simulink library "Hqaud_model_LIB_SI"  (Simulink 7.8)
settings: Solver=ode45  StartTime=0.0  StopTime=10.0  RelTol=1e-3
values from neighbouring files (symbols this model uses):
  g = 9.8065    [kostas_malakies.mat]    (also in kostas_malakies2.mat; load_PMModel.m = 9.81; main_last.m; matlab.mat)
  mass = 0.66    [kostas_malakies.mat]    (also in kostas_malakies2.mat; load_PMModel.m = 0.687; main_last.m)
  pitch_cmd2pitch_1stOrd = 1.42468924998    [kostas_malakies.mat]    (also in kostas_malakies2.mat)
  roll_cmd2roll_1stOrd = 1.38101661575    [kostas_malakies.mat]    (also in kostas_malakies2.mat)
  Td_pitch_1stOrd = 0.0601685534007    [kostas_malakies.mat]    (also in kostas_malakies2.mat)
  Td_pitch_2ndOrd = 0.0464096828042    [kostas_malakies.mat]    (also in kostas_malakies2.mat)
  Td_roll_1stOrd = 0.0529497254218    [kostas_malakies.mat]    (also in kostas_malakies2.mat)
  Td_roll_2ndOrd = 0.0402297098443    [kostas_malakies.mat]    (also in kostas_malakies2.mat)
  Td_thrust_0thOrd = 0.041    [kostas_malakies.mat]    (also in kostas_malakies2.mat)
  Td_yaw_1stOrd = 0.110660814834    [kostas_malakies.mat]    (also in kostas_malakies2.mat)
  thrust_cmd2thrust_0thOrd = 0.876575459522    [kostas_malakies.mat]    (also in kostas_malakies2.mat)
  THRUST_CMD_GAIN = -0.0835    [kostas_malakies.mat]    (also in kostas_malakies2.mat; load_PMModel.m)
  yaw_cmd2yaw_1stOrd = 2.01792090263    [kostas_malakies.mat]    (also in kostas_malakies2.mat)
libraries: cstblocks x6, Hqaud_model_LIB_SI x5, dspnetwork x2, simulink x1
settings Model: Creator=andi  LastModifiedBy=burrimi

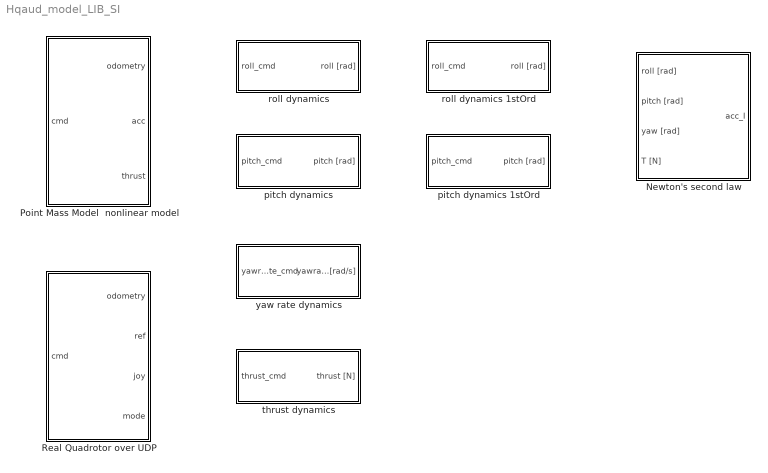
== system Hqaud_model_LIB_SI ==
  "Newton's second law  " : Subsystem
  Point Mass Model  nonlinear model : Subsystem
  Real Quadrotor over UDP : Subsystem
  "pitch dynamics  " : Subsystem
  pitch dynamics 1stOrd : Subsystem
  roll dynamics : Subsystem
  roll dynamics 1stOrd : Subsystem
  "thrust dynamics  " : Subsystem
  "yaw rate dynamics  " : Subsystem

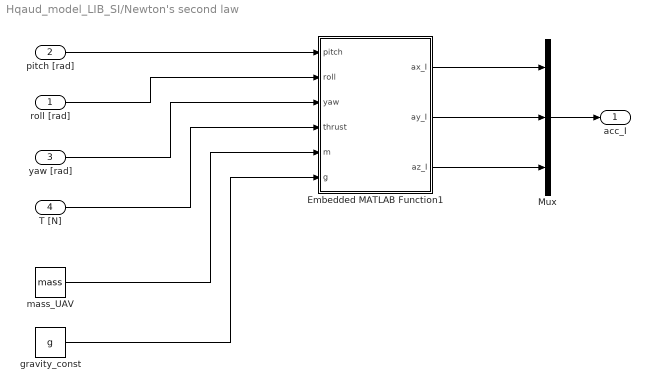
== system Hqaud_model_LIB_SI/Newton's second law   ==
  "roll [rad]  " : Inport  PortDimensions=1
  "pitch [rad]  " : Inport  Port=2  PortDimensions=1
  "yaw [rad]  " : Inport  Port=3  PortDimensions=1
  T [N] : Inport  Port=4  PortDimensions=1
  Embedded MATLAB Function1 : MATLAB Function  TreatAsAtomicUnit=on
  Mux : Mux  Inputs=3
  gravity_const : Constant  Value=g
  mass_UAV : Constant  Value=mass
  "acc_I  " : Outport  PortDimensions=3
  wires:
  Embedded MATLAB Function1/1(ax_I) -> Mux/1
  Embedded MATLAB Function1/2(ay_I) -> Mux/2
  Embedded MATLAB Function1/3(az_I) -> Mux/3
  Mux/1 -> "acc_I  "/1
  "pitch [rad]  "/1 -> Embedded MATLAB Function1/1(pitch)
  "roll [rad]  "/1 -> Embedded MATLAB Function1/2(roll)
  "yaw [rad]  "/1 -> Embedded MATLAB Function1/3(yaw)
  T [N]/1 -> Embedded MATLAB Function1/4(thrust)
  mass_UAV/1 -> Embedded MATLAB Function1/5(m)
  gravity_const/1 -> Embedded MATLAB Function1/6(g)

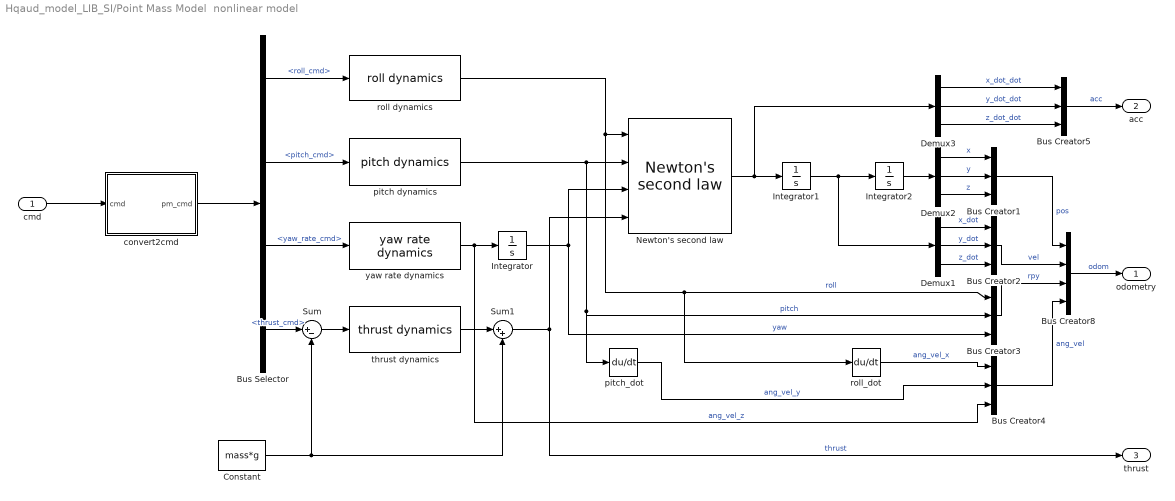
== system Hqaud_model_LIB_SI/Point Mass Model  nonlinear model ==
  cmd : Inport
  Bus Creator{1..5} (5 alike) : BusCreator  Inputs=3
  Bus Creator8 : BusCreator
  Bus Selector : BusSelector  OutputSignals=roll_cmd,pitch_cmd,yaw_rate_cmd,thrust_cmd
  Constant : Constant  Value=mass*g
  Demux1 : Demux  Outputs=3
  Demux2 : Demux  Outputs=3
  Demux3 : Demux  Outputs=3
  Integrator : Integrator
  Integrator1 : Integrator
  Integrator2 : Integrator
  "Newton's second law  " : Hqaud_model_LIB_SI/Newton's second law    SystemSampleTime=-1
  Sum : Sum  Inputs=|+-
  Sum1 : Sum  Inputs=|++
  convert2cmd : Subsystem
  "pitch dynamics  " : Hqaud_model_LIB_SI/pitch dynamics    SystemSampleTime=-1
  pitch_dot : Derivative
  roll dynamics : Hqaud_model_LIB_SI/roll dynamics  SystemSampleTime=-1
  roll_dot : Derivative
  "thrust dynamics  " : Hqaud_model_LIB_SI/thrust dynamics    SystemSampleTime=-1
  "yaw rate dynamics  " : Hqaud_model_LIB_SI/yaw rate dynamics    SystemSampleTime=-1
  odometry : Outport
  acc : Outport  Port=2
  "thrust   " : Outport  Port=3  PortDimensions=1
  wires:
  pitch_dot/1 -> Bus Creator4/2  "ang_vel_y"
  roll_dot/1 -> Bus Creator4/1  "ang_vel_x"
  Sum1/1 -> "thrust   "/1, "Newton's second law  "/4  "thrust"
  Demux3/3 -> Bus Creator5/3  "z_dot_dot"
  Demux3/2 -> Bus Creator5/2  "y_dot_dot"
  Demux3/1 -> Bus Creator5/1  "x_dot_dot"
  Bus Creator5/1 -> acc/1  "acc"
  Demux1/3 -> Bus Creator2/3  "z_dot"
  Demux1/2 -> Bus Creator2/2  "y_dot"
  Demux1/1 -> Bus Creator2/1  "x_dot"
  Demux2/1 -> Bus Creator1/1  "x"
  Demux2/3 -> Bus Creator1/3  "z"
  Bus Creator8/1 -> odometry/1  "odom"
  Bus Creator1/1 -> Bus Creator8/1  "pos"
  Bus Creator2/1 -> Bus Creator8/2  "vel"
  Bus Creator3/1 -> Bus Creator8/3  "rpy"
  Bus Creator4/1 -> Bus Creator8/4  "ang_vel"
  Bus Selector/3 -> "yaw rate dynamics  "/1  "<yaw_rate_cmd>"
  Bus Selector/2 -> "pitch dynamics  "/1  "<pitch_cmd>"
  cmd/1 -> convert2cmd/1(cmd)
  Bus Selector/4 -> Sum/1  "<thrust_cmd>"
  Sum/1 -> "thrust dynamics  "/1
  Constant/1 -> Sum1/2, Sum/2
  Demux2/2 -> Bus Creator1/2  "y"
  Integrator2/1 -> Demux2/1
  Integrator1/1 -> Demux1/1, Integrator2/1
  "Newton's second law  "/1 -> Demux3/1, Integrator1/1
  roll dynamics/1 -> roll_dot/1, Bus Creator3/1, "Newton's second law  "/1  "roll"
  "pitch dynamics  "/1 -> pitch_dot/1, Bus Creator3/2, "Newton's second law  "/2  "pitch"
  "thrust dynamics  "/1 -> Sum1/1
  Integrator/1 -> Bus Creator3/3, "Newton's second law  "/3  "yaw"
  "yaw rate dynamics  "/1 -> Bus Creator4/3, Integrator/1  "ang_vel_z"
  Bus Selector/1 -> roll dynamics/1  "<roll_cmd>"
  convert2cmd/1(pm_cmd) -> Bus Selector/1

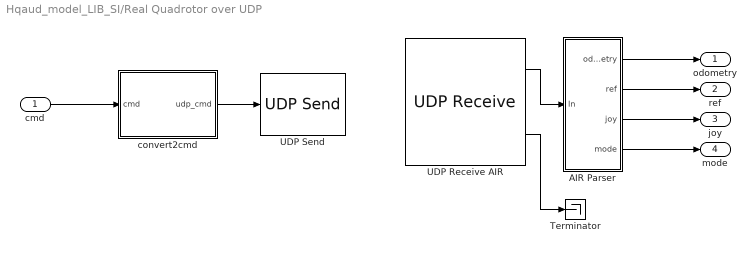
== system Hqaud_model_LIB_SI/Real Quadrotor over UDP ==
  cmd : Inport
  AIR Parser : Subsystem
  Terminator : Terminator
  UDP Receive AIR : dspnetwork/UDP Receive  localURL='0.0.0.0'  localPort=9590  remoteURL='127.0.0.1'  remotePort=-1  recvBufferSize=8192  dims=30  signalDatatype=single  isVarSize=off  showBlockingTime=on  blockingTime=0.5  sampletime=Ts  blockPlatform=LINUX
  UDP Send : dspnetwork/UDP Send  remoteURL='127.0.0.1'  remotePort=9091  localURL='255.255.255.255'  localPortSource=Automatically determine  localPort=-1  sampletime=-1  blockPlatform=LINUX  separateLengthPort=0
  convert2cmd : Subsystem
  odometry : Outport
  ref : Outport  Port=2
  joy : Outport  Port=3
  "mode   " : Outport  Port=4  PortDimensions=1
  wires:
  cmd/1 -> convert2cmd/1(cmd)
  convert2cmd/1(udp_cmd) -> UDP Send/1
  UDP Receive AIR/1 -> AIR Parser/1(In)
  AIR Parser/1(odometry) -> odometry/1
  AIR Parser/2(ref) -> ref/1
  AIR Parser/3(joy) -> joy/1
  AIR Parser/4(mode) -> "mode   "/1
  UDP Receive AIR/2 -> Terminator/1

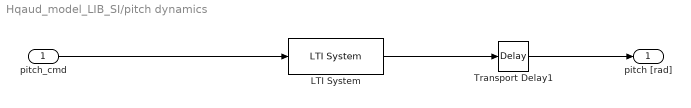
== system Hqaud_model_LIB_SI/pitch dynamics   ==
  "pitch_cmd  " : Inport  PortDimensions=1
  LTI System : cstblocks/LTI System  SystemSampleTime=-1  sys=dynamics_pitch_2ndOrd  IC=[]
  Transport Delay1 : TransportDelay  DelayTime=Td_pitch_2ndOrd  PadeOrder=delay_pade_order
  "pitch [rad] " : Outport  PortDimensions=1
  wires:
  LTI System/1 -> Transport Delay1/1
  "pitch_cmd  "/1 -> LTI System/1
  Transport Delay1/1 -> "pitch [rad] "/1

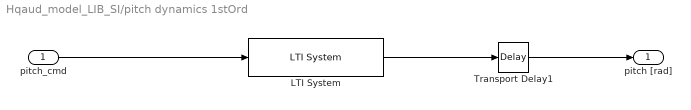
== system Hqaud_model_LIB_SI/pitch dynamics 1stOrd ==
  "pitch_cmd  " : Inport  PortDimensions=1
  LTI System : cstblocks/LTI System  SystemSampleTime=-1  sys=dynamics_pitch_1stOrd  IC=[]
  Transport Delay1 : TransportDelay  DelayTime=Td_pitch_1stOrd  PadeOrder=delay_pade_order
  "pitch [rad] " : Outport  PortDimensions=1
  wires:
  Transport Delay1/1 -> "pitch [rad] "/1
  "pitch_cmd  "/1 -> LTI System/1
  LTI System/1 -> Transport Delay1/1

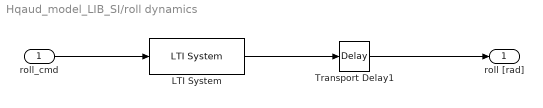
== system Hqaud_model_LIB_SI/roll dynamics ==
  "roll_cmd  " : Inport  PortDimensions=1
  LTI System : cstblocks/LTI System  SystemSampleTime=-1  sys=dynamics_roll_2ndOrd  IC=[]
  Transport Delay1 : TransportDelay  DelayTime=Td_roll_2ndOrd  PadeOrder=delay_pade_order
  "roll [rad]  " : Outport  PortDimensions=1
  wires:
  LTI System/1 -> Transport Delay1/1
  Transport Delay1/1 -> "roll [rad]  "/1
  "roll_cmd  "/1 -> LTI System/1

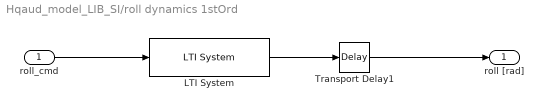
== system Hqaud_model_LIB_SI/roll dynamics 1stOrd ==
  "roll_cmd  " : Inport  PortDimensions=1
  LTI System : cstblocks/LTI System  SystemSampleTime=-1  sys=dynamics_roll_1stOrd  IC=[]
  Transport Delay1 : TransportDelay  DelayTime=Td_roll_1stOrd  PadeOrder=delay_pade_order
  "roll [rad]  " : Outport  PortDimensions=1
  wires:
  "roll_cmd  "/1 -> LTI System/1
  Transport Delay1/1 -> "roll [rad]  "/1
  LTI System/1 -> Transport Delay1/1

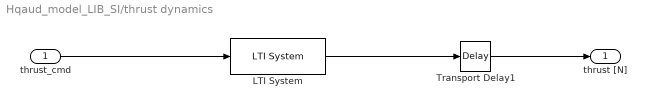
== system Hqaud_model_LIB_SI/thrust dynamics   ==
  "thrust_cmd  " : Inport  PortDimensions=1
  LTI System : cstblocks/LTI System  SystemSampleTime=-1  sys=dynamics_thrust_0thOrd  IC=[]
  Transport Delay1 : TransportDelay  DelayTime=Td_thrust_0thOrd  PadeOrder=delay_pade_order
  "thrust [N] " : Outport  PortDimensions=1
  wires:
  LTI System/1 -> Transport Delay1/1
  Transport Delay1/1 -> "thrust [N] "/1
  "thrust_cmd  "/1 -> LTI System/1

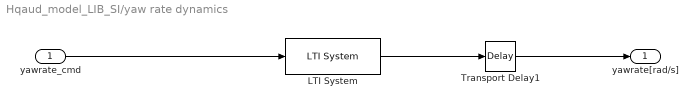
== system Hqaud_model_LIB_SI/yaw rate dynamics   ==
  "yawrate_cmd  " : Inport  PortDimensions=1
  LTI System : cstblocks/LTI System  SystemSampleTime=-1  sys=dynamics_yaw_1stOrd  IC=[]
  Transport Delay1 : TransportDelay  DelayTime=Td_yaw_1stOrd
  "yawrate[rad/s] " : Outport  PortDimensions=1
  wires:
  LTI System/1 -> Transport Delay1/1
  Transport Delay1/1 -> "yawrate[rad/s] "/1
  "yawrate_cmd  "/1 -> LTI System/1

== system Hqaud_model_LIB_SI/Point Mass Model  nonlinear model/convert2cmd ==
  cmd : Inport
  Bus Creator8 : BusCreator
  Bus Selector : BusSelector  OutputSignals=pitch_cmd,roll_cmd,thrust_cmd,yaw_rate_cmd
  pm_cmd : Outport
  wires:
  Bus Creator8/1 -> pm_cmd/1
  cmd/1 -> Bus Selector/1
  Bus Selector/1 -> Bus Creator8/1  "<pitch_cmd>"
  Bus Selector/2 -> Bus Creator8/2  "<roll_cmd>"
  Bus Selector/4 -> Bus Creator8/4  "<yaw_rate_cmd>"
  Bus Selector/3 -> Bus Creator8/3  "<thrust_cmd>"

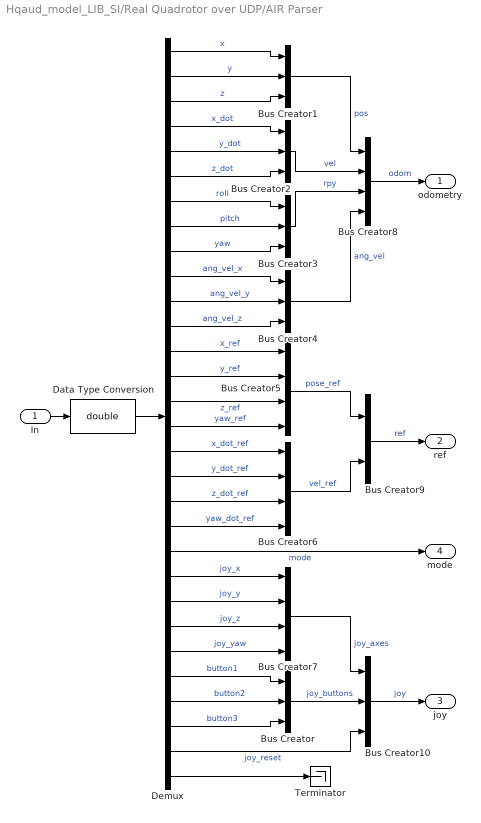
== system Hqaud_model_LIB_SI/Real Quadrotor over UDP/AIR Parser ==
  In : Inport
  Bus Creator{,1..4,10} (6 alike) : BusCreator  Inputs=3
  Bus Creator{5..8} (4 alike) : BusCreator
  Bus Creator9 : BusCreator  Inputs=2
  Data Type Conversion : DataTypeConversion  OutDataTypeStr=double
  Demux : Demux  Outputs=30
  Terminator : Terminator
  odometry : Outport
  ref : Outport  Port=2
  joy : Outport  Port=3
  mode : Outport  Port=4
  wires:
  In/1 -> Data Type Conversion/1
  Data Type Conversion/1 -> Demux/1
  Demux/1 -> Bus Creator1/1  "x"
  Demux/7 -> Bus Creator3/1  "roll"
  Demux/8 -> Bus Creator3/2  "pitch"
  Demux/9 -> Bus Creator3/3  "yaw"
  Demux/15 -> Bus Creator5/3  "z_ref"
  Demux/14 -> Bus Creator5/2  "y_ref"
  Demux/13 -> Bus Creator5/1  "x_ref"
  Demux/16 -> Bus Creator5/4  "yaw_ref"
  Demux/2 -> Bus Creator1/2  "y"
  Demux/3 -> Bus Creator1/3  "z"
  Demux/4 -> Bus Creator2/1  "x_dot"
  Demux/5 -> Bus Creator2/2  "y_dot"
  Demux/6 -> Bus Creator2/3  "z_dot"
  Demux/19 -> Bus Creator6/3  "z_dot_ref"
  Demux/18 -> Bus Creator6/2  "y_dot_ref"
  Demux/17 -> Bus Creator6/1  "x_dot_ref"
  Demux/20 -> Bus Creator6/4  "yaw_dot_ref"
  Demux/12 -> Bus Creator4/3  "ang_vel_z"
  Demux/11 -> Bus Creator4/2  "ang_vel_y"
  Demux/10 -> Bus Creator4/1  "ang_vel_x"
  Demux/21 -> mode/1  "mode"
  Bus Creator5/1 -> Bus Creator9/1  "pose_ref"
  Bus Creator6/1 -> Bus Creator9/2  "vel_ref"
  Demux/22 -> Bus Creator7/1  "joy_x"
  Demux/23 -> Bus Creator7/2  "joy_y"
  Demux/24 -> Bus Creator7/3  "joy_z"
  Demux/25 -> Bus Creator7/4  "joy_yaw"
  Bus Creator7/1 -> Bus Creator10/1  "joy_axes"
  Demux/26 -> Bus Creator/1  "button1"
  Demux/28 -> Bus Creator/3  "button3"
  Demux/27 -> Bus Creator/2  "button2"
  Bus Creator/1 -> Bus Creator10/2  "joy_buttons"
  Bus Creator4/1 -> Bus Creator8/4  "ang_vel"
  Bus Creator3/1 -> Bus Creator8/3  "rpy"
  Bus Creator2/1 -> Bus Creator8/2  "vel"
  Bus Creator1/1 -> Bus Creator8/1  "pos"
  Demux/29 -> Bus Creator10/3  "joy_reset"
  Bus Creator10/1 -> joy/1  "joy"
  Bus Creator9/1 -> ref/1  "ref"
  Bus Creator8/1 -> odometry/1  "odom"
  Demux/30 -> Terminator/1

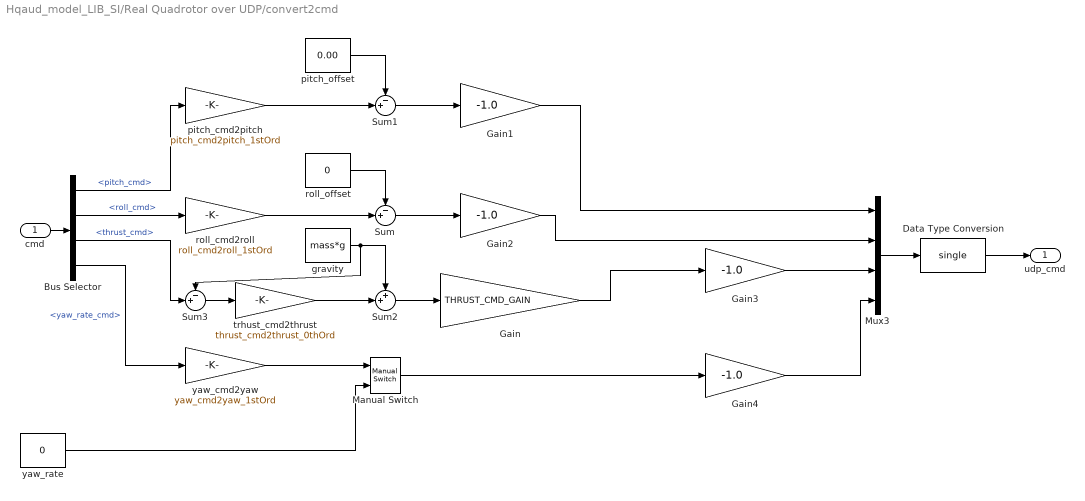
== system Hqaud_model_LIB_SI/Real Quadrotor over UDP/convert2cmd ==
  cmd : Inport
  Bus Selector : BusSelector  OutputSignals=pitch_cmd,roll_cmd,thrust_cmd,yaw_rate_cmd
  Data Type Conversion : DataTypeConversion  OutDataTypeStr=single
  Gain : Gain  Gain=THRUST_CMD_GAIN
  Gain{1..4} (4 alike) : Gain  Gain=-1.0
  Manual Switch : simulink/Signal Routing/Manual Switch  SystemSampleTime=-1  sw=1  action=0  varsize=off
  Mux3 : Mux
  Sum : Sum  Inputs=-+|
  Sum1 : Sum  Inputs=-+|
  Sum2 : Sum  Inputs=++|
  Sum3 : Sum  Inputs=-+|
  gravity : Constant  Value=mass*g
  pitch_cmd2pitch : Gain  Gain=pitch_cmd2pitch_1stOrd
  pitch_offset : Constant  Value=0.00
  roll_cmd2roll : Gain  Gain=roll_cmd2roll_1stOrd
  roll_offset : Constant  Value=0
  trhust_cmd2thrust : Gain  Gain=thrust_cmd2thrust_0thOrd
  yaw_cmd2yaw : Gain  Gain=yaw_cmd2yaw_1stOrd
  yaw_rate : Constant  Value=0
  udp_cmd : Outport
  wires:
  Gain4/1 -> Mux3/4
  Gain3/1 -> Mux3/3
  Gain2/1 -> Mux3/2
  Gain/1 -> Gain3/1
  Gain1/1 -> Mux3/1
  pitch_offset/1 -> Sum1/1
  Sum1/1 -> Gain1/1
  roll_offset/1 -> Sum/1
  Sum/1 -> Gain2/1
  Mux3/1 -> Data Type Conversion/1
  Data Type Conversion/1 -> udp_cmd/1
  gravity/1 -> Sum2/1, Sum3/1
  Sum2/1 -> Gain/1
  Manual Switch/1 -> Gain4/1
  yaw_rate/1 -> Manual Switch/2
  cmd/1 -> Bus Selector/1
  Bus Selector/1 -> pitch_cmd2pitch/1  "<pitch_cmd>"
  Bus Selector/2 -> roll_cmd2roll/1  "<roll_cmd>"
  yaw_cmd2yaw/1 -> Manual Switch/1
  trhust_cmd2thrust/1 -> Sum2/2
  pitch_cmd2pitch/1 -> Sum1/2
  roll_cmd2roll/1 -> Sum/2
  Bus Selector/3 -> Sum3/2  "<thrust_cmd>"
  Sum3/1 -> trhust_cmd2thrust/1
  Bus Selector/4 -> yaw_cmd2yaw/1  "<yaw_rate_cmd>"

== matlab function Newton's second law /Embedded MATLAB Function1 ==
  data: pitch input double; ax_I output double; roll input double; yaw input double; thrust input double; m input double; g input double; ay_I output double; az_I output double
function [ax_I, ay_I, az_I] = fcn(pitch, roll, yaw, thrust, m, g)
%#eml

acc = -thrust/m*[ cos(yaw)*sin(pitch)*cos(roll)+sin(yaw)*sin(roll);...
                sin(yaw)*sin(pitch)*cos(roll)-cos(yaw)*sin(roll);...
                cos(pitch)*cos(roll)]...
             +[ 0; 0; g ];
         
ax_I = acc(1);
ay_I = acc(2);
az_I = acc(3);
